simulink model "robot_controller"  (R2020b)
settings: Solver=VariableStepAuto  StartTime=0.0  StopTime=Inf  RelTol=1e-3
undefined symbols (not defined in the file): f
libraries: simulink x1, fuzblock x1, sldrtlib x1, instrumentlib x1, dspnetwork x1
settings Model: Creator=48796  LastModifiedBy=48796
settings SFSimCC: CustomCodeUndefinedFunction=UseInterfaceOnly

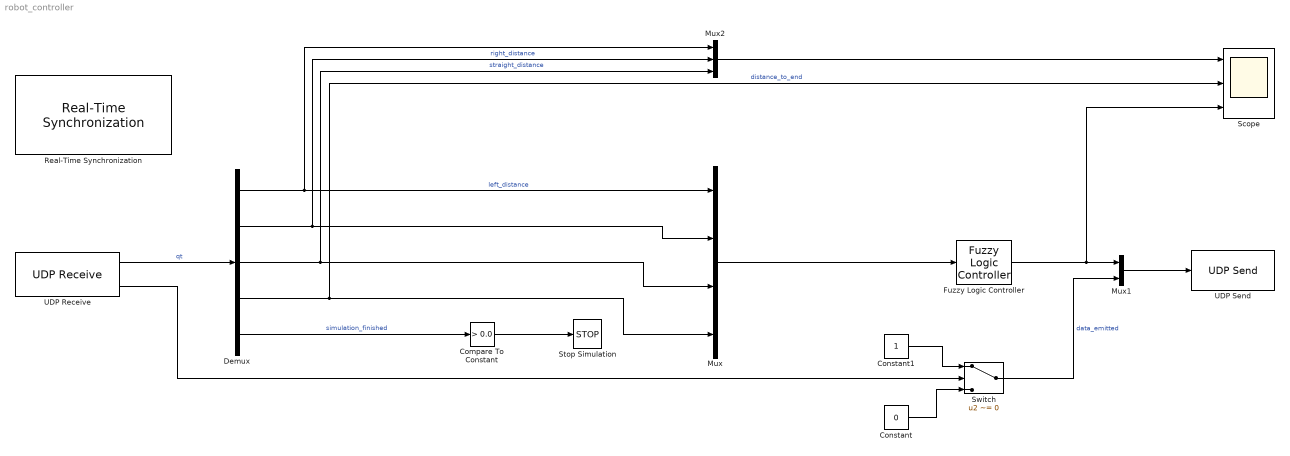
== system robot_controller ==
  Compare To Constant : simulink/Logic and Bit Operations/Compare To Constant  relop=>  const=0.0  OutDataTypeStr=boolean
  Constant : Constant  Value=0
  Constant1 : Constant
  Demux : Demux  Outputs=5
  Fuzzy Logic Controller : fuzblock/Fuzzy Logic  Controller  FIS='r5.fis'  OutputSampleNumber=101  DataType=double  FuzzifiedInputs=off  RuleFiringStrengths=off  RuleOutputs=off  AggregatedOutputs=off  SimulateUsing=Interpreted execution  OutOfRangeInputValueMessage=warning  NoRuleFiredMessage=warning  EmptyOutputFuzzySetMessage=warning
  Mux : Mux
  Mux1 : Mux  Inputs=2
  Mux2 : Mux  Inputs=3
  Real-Time Synchronization : sldrtlib/Real-Time Synchronization  SampleTime=0.1  MaxMissedTicks=100000  ShowMissedTicks=off  YieldWhenWaiting=off
  Scope : Scope  NumInputPorts=3
  Stop Simulation : Stop
  Switch : Switch  Criteria=u2 ~= 0
  UDP Receive : instrumentlib/UDP Receive  Host=localhost  Port=9090  LocalPort=7777  EnablePortSharing=off  GetLatestData=off  DataSize="[1  5]"  DataType=double  ASCIIFormatting=%f,  Terminator=LF  ByteOrder=BigEndian  EnableBlockingMode=off  Timeout=10  SampleTime=0.1  LocalAddress=192.168.100.212
  UDP Send : dspnetwork/UDP Send  remoteURL='192.168.100.1'  remotePort=2137  localURL='0.0.0.0'  localPortSource=Automatically determine  localPort=-1  sendBufferSize=8192  sampletime=-1  blockPlatform=[]  separateLengthPort=0
  wires:
  Mux/1 -> Fuzzy Logic Controller/1
  UDP Receive/1 -> Demux/1  "qt"
  Demux/5 -> Compare To Constant/1  "simulation_finished"
  Demux/1 -> Mux2/1, Mux/1  "left_distance"
  Demux/2 -> Mux2/2, Mux/2  "right_distance"
  Demux/3 -> Mux2/3, Mux/3  "straight_distance"
  Demux/4 -> Scope/2, Mux/4  "distance_to_end"
  Compare To Constant/1 -> Stop Simulation/1
  Fuzzy Logic Controller/1 -> Scope/3, Mux1/1
  Switch/1 -> Mux1/2  "data_emitted"
  Constant1/1 -> Switch/1
  Constant/1 -> Switch/3
  UDP Receive/2 -> Switch/2
  Mux2/1 -> Scope/1
  Mux1/1 -> UDP Send/1
